simulink model "Multi_FW_formation_control_wind"  (R2023b)
settings: Solver=FixedStepAuto  StartTime=0.0  StopTime=70  FixedStep=0.001  RelTol=1e-3
undefined symbols (not defined in the file or in its folder): fc, hc, lc
libraries: Fixed_Wing x4, simulink x1
settings Model: Creator=TigerWuu  LastModifiedBy=NCS
settings SolverCC: MaxConsecutiveMinStep=10  ZeroCrossAlgorithm=Adaptive  EnableFixedStepZeroCrossing=on
settings OptimizationCC: EnhancedBackFolding=on  PassReuseOutputArgsAs=Individual arguments  ZeroExternalMemoryAtStartup=off  ZeroInternalMemoryAtStartup=off  MaxStackSize=64  OptimizeBlockOrder=speed  DifferentSizesBufferReuse=on  OptimizationCustomize=off  EfficientTunableParamExpr=on
settings DebuggingCC: IgnoredZcDiagnostic=none  ParameterTunabilityLossMsg=error  UnconnectedInputMsg=warning  UnconnectedOutputMsg=warning  UnconnectedLineMsg=warning  UnderSpecifiedDimensionMsg=warning
settings HardwareCC: UseEmbeddedCoderFeatures=off
settings ModelReferenceCC: EnableRefExpFcnMdlSchedulingChecks=on
settings SFSimCC: MATLABDynamicMemAlloc=off
settings RTWCC: Description=Embedded Coder  SystemTargetFile=ert.tlc  HardwareBoard=Robot Operating System 2 (ROS 2)  TLCOptions="-aInlineSetEventsForThisBaseRateFcn=TLC_FALSE -aSuppressMultiTaskScheduler=TLC_FALSE  -aRateBasedStepFcn=0"  TemplateMakefile=ert_default_tmf  Toolchain=Colcon Tools  TargetLang=C++  DLArmComputeVersion=19.05
settings CodeAppCC: ForceParamTrailComments=on  IgnoreCustomStorageClasses=off  OperatorAnnotations=on  SimulinkDataObjDesc=on  SFDataObjDesc=on  InsertBlockDesc=on
settings ERTTargetCC: CodeInterfacePackaging=C++ class  SupportNonInlinedSFcns=on  RootIOFormat=Structure reference

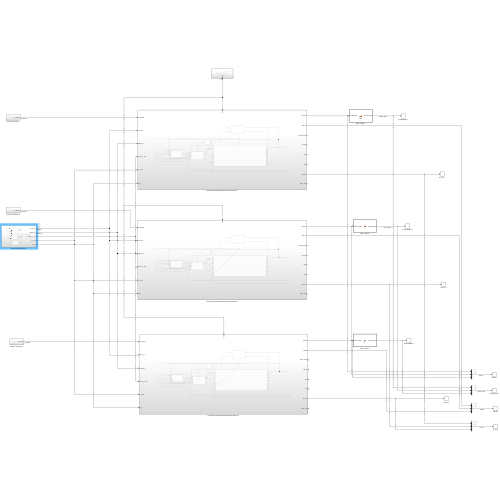
[thumbnail: Simulink's stored preview of the top-level diagram]
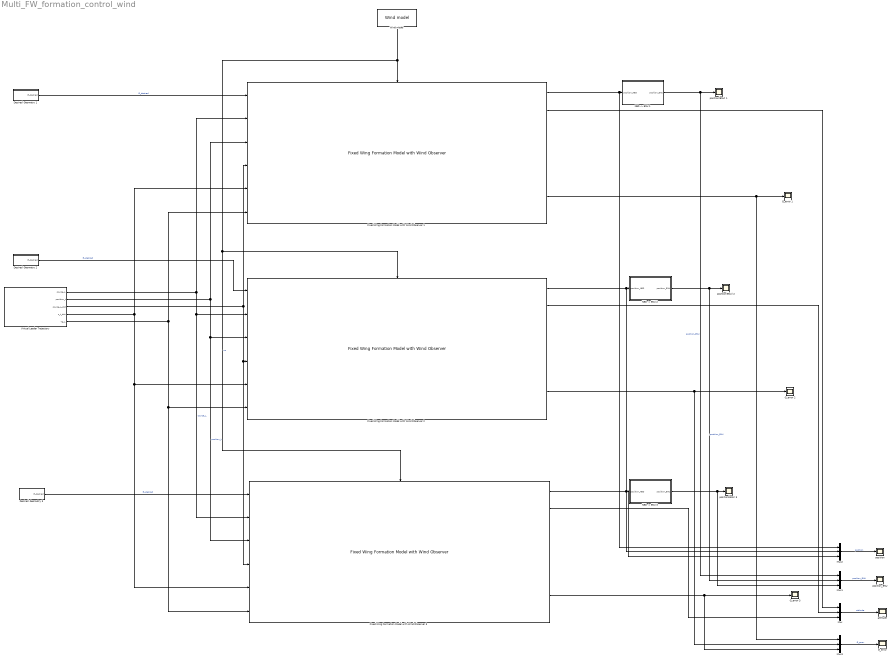
== system Multi_FW_formation_control_wind ==
  Desired  Geometry 1 : Subsystem
  Desired  Geometry 2 : Subsystem
  Desired  Geometry 3 : Subsystem
  Fixed Wing Formation Model with Wind Observer 1 : Fixed_Wing/Fixed Wing Formation Model with Wind Observer  SystemSampleTime=-1  VariantActivationTime=update diagram  AllowFlexibleInterface=on  Latency=0  AutoFrameSizeCalculation=off
      settings: SourceProductName=Fixed-Wing Model  PortSchema="{\"entries\":[{\"content\":{\"sides\":[{\"content\":{\"connectorIds\":[\"In1\",\"In2\",\"In3\",\"In4\",\"In5\",\"In6\"]},\"type\":\"ConnectorPlacement.EquallySpacedRectSide\",\"uuid\":\"527b8280-b7bb-4bbf-b75e-797629a1d02f\"},{\"content\":{\"connectorIds\":[\"Out1\",\"Out2\",\"Out3\",\"Out4\",\"Out5\",\"Out6\",\"Out7\",\"Out8\"],\"side\":\"RIGHT\"},\"type\":\"ConnectorPlacement.EquallySpacedRectSide\",\"uuid\":\"83651618-4cce-4797-8c5d-5752aadadd0e\"},{\"content\":{\"connectorIds\":[\"In7\"],\"side\":\"TOP\"},\"type\":\"ConnectorPlacement.EquallySpacedRectSide\",\"uuid\":\"91f129b3-c1c6-46ff-9e73-d368da7d167a\"}]},\"type\":\"ConnectorPlacement.EquallySpacedConnector\",\"uuid\":\"d5eae0c8-1f9e-4313-b74c-0f7e22e43491\"}],\"packageUris\":[\"http://schema.mathworks.com/mf0/Connector/R2020b\"],\"version\":\"1.0\"}"
  Fixed Wing Formation Model with Wind Observer 2 : Fixed_Wing/Fixed Wing Formation Model with Wind Observer  SystemSampleTime=-1  VariantActivationTime=update diagram  AllowFlexibleInterface=on  Latency=0  AutoFrameSizeCalculation=off
      settings: SourceProductName=Fixed-Wing Model  PortSchema="{\"entries\":[{\"content\":{\"sides\":[{\"content\":{\"connectorIds\":[\"In1\",\"In2\",\"In3\",\"In4\",\"In5\",\"In6\"]},\"type\":\"ConnectorPlacement.EquallySpacedRectSide\",\"uuid\":\"527b8280-b7bb-4bbf-b75e-797629a1d02f\"},{\"content\":{\"connectorIds\":[\"Out1\",\"Out2\",\"Out3\",\"Out4\",\"Out5\",\"Out6\",\"Out7\",\"Out8\"],\"side\":\"RIGHT\"},\"type\":\"ConnectorPlacement.EquallySpacedRectSide\",\"uuid\":\"83651618-4cce-4797-8c5d-5752aadadd0e\"},{\"content\":{\"connectorIds\":[\"In7\"],\"side\":\"TOP\"},\"type\":\"ConnectorPlacement.EquallySpacedRectSide\",\"uuid\":\"91f129b3-c1c6-46ff-9e73-d368da7d167a\"}]},\"type\":\"ConnectorPlacement.EquallySpacedConnector\",\"uuid\":\"d5eae0c8-1f9e-4313-b74c-0f7e22e43491\"}],\"packageUris\":[\"http://schema.mathworks.com/mf0/Connector/R2020b\"],\"version\":\"1.0\"}"
  Fixed Wing Formation Model with Wind Observer 3 : Fixed_Wing/Fixed Wing Formation Model with Wind Observer  SystemSampleTime=-1  VariantActivationTime=update diagram  AllowFlexibleInterface=on  Latency=0  AutoFrameSizeCalculation=off
      settings: SourceProductName=Fixed-Wing Model  PortSchema="{\"entries\":[{\"content\":{\"sides\":[{\"content\":{\"connectorIds\":[\"In1\",\"In2\",\"In3\",\"In4\",\"In5\",\"In6\"]},\"type\":\"ConnectorPlacement.EquallySpacedRectSide\",\"uuid\":\"527b8280-b7bb-4bbf-b75e-797629a1d02f\"},{\"content\":{\"connectorIds\":[\"Out1\",\"Out2\",\"Out3\",\"Out4\",\"Out5\",\"Out6\",\"Out7\",\"Out8\"],\"side\":\"RIGHT\"},\"type\":\"ConnectorPlacement.EquallySpacedRectSide\",\"uuid\":\"83651618-4cce-4797-8c5d-5752aadadd0e\"},{\"content\":{\"connectorIds\":[\"In7\"],\"side\":\"TOP\"},\"type\":\"ConnectorPlacement.EquallySpacedRectSide\",\"uuid\":\"91f129b3-c1c6-46ff-9e73-d368da7d167a\"}]},\"type\":\"ConnectorPlacement.EquallySpacedConnector\",\"uuid\":\"d5eae0c8-1f9e-4313-b74c-0f7e22e43491\"}],\"packageUris\":[\"http://schema.mathworks.com/mf0/Connector/R2020b\"],\"version\":\"1.0\"}"
  G_error : Scope
  G_error 1 : Scope
  G_error 2 : Scope
  G_error 3 : Scope
  Mux{,1..3} (4 alike) : Mux  Inputs=3
  "NED -> ENU 1" : MATLAB Function  TreatAsAtomicUnit=on
  "NED -> ENU 2" : MATLAB Function  TreatAsAtomicUnit=on
  "NED -> ENU 3" : MATLAB Function  TreatAsAtomicUnit=on
  Virtual Leader Trajectory : Subsystem
  Wind model : Fixed_Wing/Wind model  SystemSampleTime=-1  VariantActivationTime=update diagram  AllowFlexibleInterface=on  Latency=0  AutoFrameSizeCalculation=off
      settings: SourceProductName=Fixed-Wing Model  PortSchema="{\"entries\":[{\"content\":{\"sides\":[{\"content\":{},\"type\":\"ConnectorPlacement.EquallySpacedRectSide\",\"uuid\":\"19ef0eb7-c626-45ec-b76b-8668fc024824\"},{\"content\":{\"side\":\"RIGHT\"},\"type\":\"ConnectorPlacement.EquallySpacedRectSide\",\"uuid\":\"89e72569-ab94-4162-a6e2-b425ef08f724\"},{\"content\":{\"side\":\"TOP\"},\"type\":\"ConnectorPlacement.EquallySpacedRectSide\",\"uuid\":\"6d9409e9-6822-4cd9-902f-e5665cb68433\"},{\"content\":{\"connectorIds\":[\"Out1\"],\"side\":\"BOTTOM\"},\"type\":\"ConnectorPlacement.EquallySpacedRectSide\",\"uuid\":\"39a83352-0924-44fa-be5d-94a7c28bbbf3\"}]},\"type\":\"ConnectorPlacement.EquallySpacedConnector\",\"uuid\":\"6cf6ae00-ef23-42a2-99b2-ca60e191fb03\"}],\"packageUris\":[\"http://schema.mathworks.com/mf0/Connector/R2020b\"],\"version\":\"1.0\"}"
  attitude : Scope
  position : Scope
  position(ENU) 1 : Scope
  position(ENU) 2 : Scope
  position(ENU) 3 : Scope
  position_ENU : Scope
  wires:
  "NED -> ENU 1"/1(position_ENU) -> Mux1/1, position(ENU) 1/1  "position_ENU"
  Desired  Geometry 1/1(G_desired) -> Fixed Wing Formation Model with Wind Observer 1/1  "G_desired"
  Virtual Leader Trajectory/1(course_L) -> Fixed Wing Formation Model with Wind Observer 2/2, Fixed Wing Formation Model with Wind Observer 3/2, Fixed Wing Formation Model with Wind Observer 1/2  "course_L"
  Virtual Leader Trajectory/2(position_L) -> Fixed Wing Formation Model with Wind Observer 2/3, Fixed Wing Formation Model with Wind Observer 3/3, Fixed Wing Formation Model with Wind Observer 1/3  "position_L"
  Virtual Leader Trajectory/3(course_L_dot) -> Fixed Wing Formation Model with Wind Observer 2/4, Fixed Wing Formation Model with Wind Observer 3/4, Fixed Wing Formation Model with Wind Observer 1/4
  Virtual Leader Trajectory/4(z_L_dot) -> Fixed Wing Formation Model with Wind Observer 2/5, Fixed Wing Formation Model with Wind Observer 3/5, Fixed Wing Formation Model with Wind Observer 1/5
  Virtual Leader Trajectory/5(Vg_L) -> Fixed Wing Formation Model with Wind Observer 2/6, Fixed Wing Formation Model with Wind Observer 3/6, Fixed Wing Formation Model with Wind Observer 1/6
  Wind model/1 -> Fixed Wing Formation Model with Wind Observer 1/7, Fixed Wing Formation Model with Wind Observer 2/7, Fixed Wing Formation Model with Wind Observer 3/7  "ws"
  Fixed Wing Formation Model with Wind Observer 1/1 -> Mux2/1, "NED -> ENU 1"/1(position_NED)
  Desired  Geometry 2/1(G_desired) -> Fixed Wing Formation Model with Wind Observer 2/1  "G_desired"
  "NED -> ENU 2"/1(position_ENU) -> Mux1/2, position(ENU) 2/1  "position_ENU"
  Fixed Wing Formation Model with Wind Observer 2/1 -> Mux2/2, "NED -> ENU 2"/1(position_NED)
  Fixed Wing Formation Model with Wind Observer 2/7 -> Mux3/2, G_error 2/1
  Desired  Geometry 3/1(G_desired) -> Fixed Wing Formation Model with Wind Observer 3/1  "G_desired"
  "NED -> ENU 3"/1(position_ENU) -> Mux1/3, position(ENU) 3/1
  Fixed Wing Formation Model with Wind Observer 3/1 -> Mux2/3, "NED -> ENU 3"/1(position_NED)
  Fixed Wing Formation Model with Wind Observer 3/7 -> Mux3/3, G_error 3/1
  Fixed Wing Formation Model with Wind Observer 1/2 -> Mux/1
  Fixed Wing Formation Model with Wind Observer 2/2 -> Mux/2
  Fixed Wing Formation Model with Wind Observer 3/2 -> Mux/3
  Fixed Wing Formation Model with Wind Observer 1/7 -> Mux3/1, G_error 1/1
  Mux2/1 -> position/1  "position"
  Mux1/1 -> position_ENU/1  "position_ENU"
  Mux/1 -> attitude/1  "attitude"
  Mux3/1 -> G_error/1  "G_error"

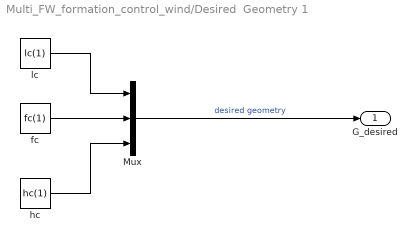
== system Multi_FW_formation_control_wind/Desired  Geometry 1 ==
  Mux : Mux  Inputs=3
  fc : Constant  Value=fc(1)
  hc : Constant  Value=hc(1)
  lc : Constant  Value=lc(1)
  G_desired : Outport
  wires:
  Mux/1 -> G_desired/1  "desired geometry"
  lc/1 -> Mux/1
  fc/1 -> Mux/2
  hc/1 -> Mux/3

== system Multi_FW_formation_control_wind/Desired  Geometry 2 ==
  Mux : Mux  Inputs=3
  fc : Constant  Value=fc(2)
  hc : Constant  Value=hc(2)
  lc : Constant  Value=lc(2)
  G_desired : Outport
  wires:
  Mux/1 -> G_desired/1  "desired geometry"
  lc/1 -> Mux/1
  fc/1 -> Mux/2
  hc/1 -> Mux/3

== system Multi_FW_formation_control_wind/Desired  Geometry 3 ==
  Mux : Mux  Inputs=3
  fc : Constant  Value=fc(3)
  hc : Constant  Value=hc(3)
  lc : Constant  Value=lc(3)
  G_desired : Outport
  wires:
  Mux/1 -> G_desired/1  "desired geometry"
  lc/1 -> Mux/1
  fc/1 -> Mux/2
  hc/1 -> Mux/3

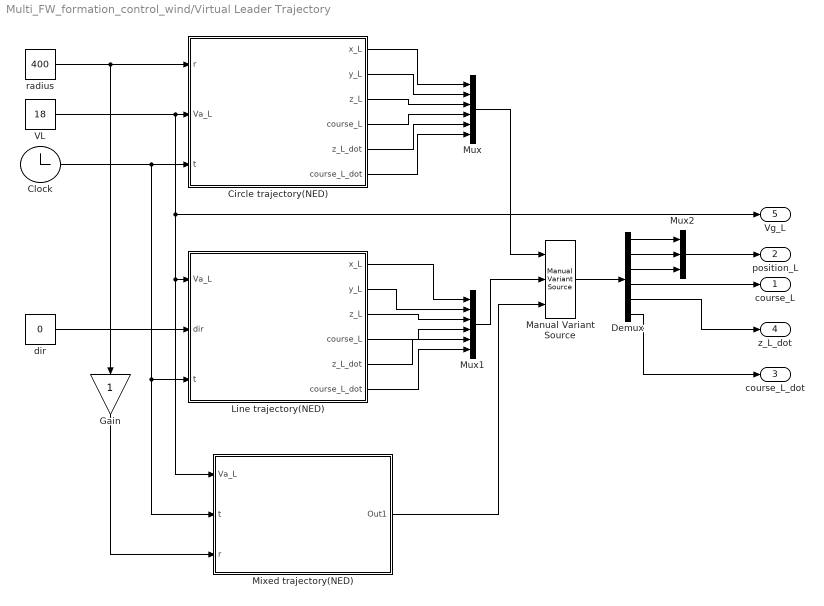
== system Multi_FW_formation_control_wind/Virtual Leader Trajectory ==
  Circle trajectory(NED) : MATLAB Function  TreatAsAtomicUnit=on
  Clock : Clock
  Demux : Demux  Outputs=6
  Gain : Gain
  Line trajectory(NED) : MATLAB Function  TreatAsAtomicUnit=on
  Manual Variant Source : simulink/Signal Routing/Manual Variant Source  NumChoices=3  LabelModeActiveChoice=V_2
  Mixed trajectory(NED) : Subsystem
  Mux : Mux  Inputs=6
  Mux1 : Mux  Inputs=6
  Mux2 : Mux  Inputs=3
  VL : Constant  Value=18
  dir : Constant  Value=0
  radius : Constant  Value=400
  course_L : Outport
  position_L : Outport  Port=2
  course_L_dot : Outport  Port=3
  z_L_dot : Outport  Port=4
  Vg_L : Outport  Port=5
  wires:
  radius/1 -> Circle trajectory(NED)/1(r), Gain/1
  VL/1 -> Vg_L/1, Mixed trajectory(NED)/1(Va_L), Line trajectory(NED)/1(Va_L), Circle trajectory(NED)/2(Va_L)
  Clock/1 -> Mixed trajectory(NED)/2(t), Line trajectory(NED)/3(t), Circle trajectory(NED)/3(t)
  Mux/1 -> Manual Variant Source/1
  Circle trajectory(NED)/1(x_L) -> Mux/1
  Circle trajectory(NED)/2(y_L) -> Mux/2
  Circle trajectory(NED)/3(z_L) -> Mux/3
  Line trajectory(NED)/1(x_L) -> Mux1/1
  Line trajectory(NED)/2(y_L) -> Mux1/2
  Line trajectory(NED)/3(z_L) -> Mux1/3
  Line trajectory(NED)/4(course_L) -> Mux1/4
  Mux1/1 -> Manual Variant Source/2
  Manual Variant Source/1 -> Demux/1
  Demux/1 -> Mux2/1
  Demux/2 -> Mux2/2
  Demux/3 -> Mux2/3
  Mux2/1 -> position_L/1
  Circle trajectory(NED)/6(course_L_dot) -> Mux/6
  Line trajectory(NED)/6(course_L_dot) -> Mux1/6
  Line trajectory(NED)/5(z_L_dot) -> Mux1/5
  Demux/4 -> course_L/1
  Demux/5 -> z_L_dot/1
  Demux/6 -> course_L_dot/1
  Circle trajectory(NED)/4(course_L) -> Mux/4
  Circle trajectory(NED)/5(z_L_dot) -> Mux/5
  Gain/1 -> Mixed trajectory(NED)/3(r)
  Mixed trajectory(NED)/1(Out1) -> Manual Variant Source/3
  dir/1 -> Line trajectory(NED)/2(dir)

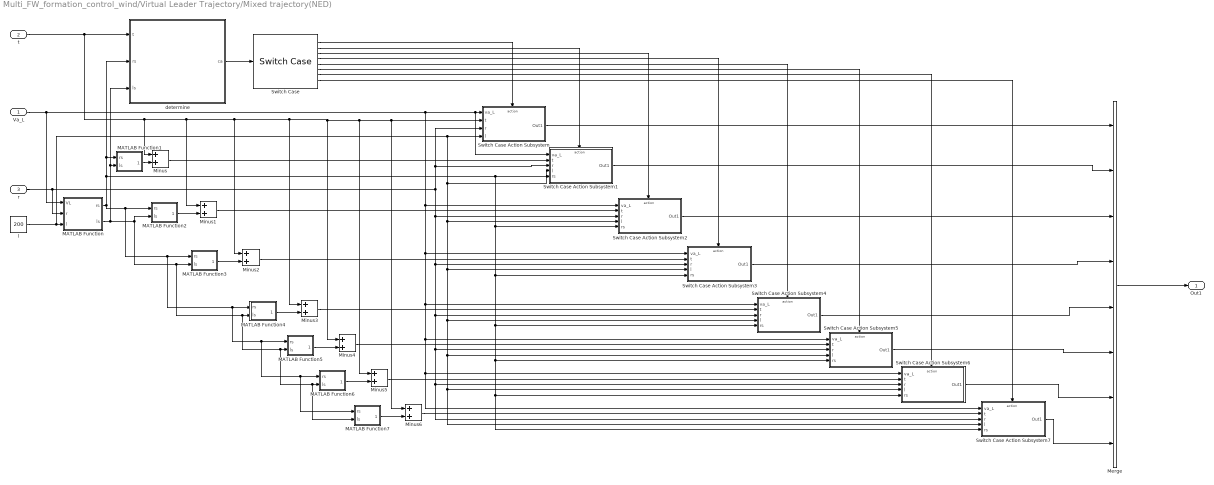
== system Multi_FW_formation_control_wind/Virtual Leader Trajectory/Mixed trajectory(NED) ==
  Va_L : Inport
  t : Inport  Port=2
  r : Inport  Port=3
  MATLAB Function : MATLAB Function  TreatAsAtomicUnit=on
  MATLAB Function1 : MATLAB Function  TreatAsAtomicUnit=on
  MATLAB Function2 : MATLAB Function  TreatAsAtomicUnit=on
  MATLAB Function3 : MATLAB Function  TreatAsAtomicUnit=on
  MATLAB Function4 : MATLAB Function  TreatAsAtomicUnit=on
  MATLAB Function5 : MATLAB Function  TreatAsAtomicUnit=on
  MATLAB Function6 : MATLAB Function  TreatAsAtomicUnit=on
  MATLAB Function7 : MATLAB Function  TreatAsAtomicUnit=on
  Merge : Merge  Inputs=8
  Minus{,1..6} (7 alike) : Sum
  Switch Case : SwitchCase  CaseConditions={1,2,3,4,5,6,7,8}  ShowDefaultCase=off
  Switch Case Action Subsystem : Subsystem  TreatAsAtomicUnit=on
  Switch Case Action Subsystem1 : Subsystem  TreatAsAtomicUnit=on
  Switch Case Action Subsystem2 : Subsystem  TreatAsAtomicUnit=on
  Switch Case Action Subsystem3 : Subsystem  TreatAsAtomicUnit=on
  Switch Case Action Subsystem4 : Subsystem  TreatAsAtomicUnit=on
  Switch Case Action Subsystem5 : Subsystem  TreatAsAtomicUnit=on
  Switch Case Action Subsystem6 : Subsystem  TreatAsAtomicUnit=on
  Switch Case Action Subsystem7 : Subsystem  TreatAsAtomicUnit=on
  determine : MATLAB Function  TreatAsAtomicUnit=on
  l : Constant  Value=200
  Out1 : Outport
  wires:
  determine/1(ca) -> Switch Case/1
  Switch Case/1 -> Switch Case Action Subsystem/Action
  MATLAB Function1/1(offset) -> Minus/2
  Switch Case/2 -> Switch Case Action Subsystem1/Action
  r/1 -> Switch Case Action Subsystem6/3(r), Switch Case Action Subsystem7/3(r), Switch Case Action Subsystem5/3(r), Switch Case Action Subsystem4/3(r), Switch Case Action Subsystem3/3(r), Switch Case Action Subsystem2/3(r), Switch Case Action Subsystem/3(r), Switch Case Action Subsystem1/3(r), MATLAB Function/2(r)
  MATLAB Function2/1(offset) -> Minus1/2
  Minus1/1 -> Switch Case Action Subsystem2/2(t)
  Switch Case/3 -> Switch Case Action Subsystem2/Action
  Switch Case/4 -> Switch Case Action Subsystem3/Action
  Minus/1 -> Switch Case Action Subsystem1/2(t)
  MATLAB Function3/1(offset) -> Minus2/2
  Minus2/1 -> Switch Case Action Subsystem3/2(t)
  Va_L/1 -> Switch Case Action Subsystem1/1(va_L), Switch Case Action Subsystem/1(va_L), Switch Case Action Subsystem4/1(va_L), Switch Case Action Subsystem5/1(va_L), Switch Case Action Subsystem6/1(va_L), Switch Case Action Subsystem7/1(va_L), Switch Case Action Subsystem3/1(va_L), Switch Case Action Subsystem2/1(va_L), MATLAB Function/1(VL)
  Minus3/1 -> Switch Case Action Subsystem4/2(t)
  Switch Case/5 -> Switch Case Action Subsystem4/Action
  MATLAB Function4/1(offset) -> Minus3/2
  Switch Case/6 -> Switch Case Action Subsystem5/Action
  MATLAB Function5/1(offset) -> Minus4/2
  Minus4/1 -> Switch Case Action Subsystem5/2(t)
  Switch Case/7 -> Switch Case Action Subsystem6/Action
  MATLAB Function6/1(offset) -> Minus5/2
  Minus5/1 -> Switch Case Action Subsystem6/2(t)
  Switch Case/8 -> Switch Case Action Subsystem7/Action
  t/1 -> Minus/1, Minus1/1, Minus2/1, Minus3/1, Minus4/1, Minus5/1, Minus6/1, Switch Case Action Subsystem/2(t), determine/1(t)
  Minus6/1 -> Switch Case Action Subsystem7/2(t)
  MATLAB Function7/1(offset) -> Minus6/2
  Switch Case Action Subsystem/1(Out1) -> Merge/1
  Switch Case Action Subsystem1/1(Out1) -> Merge/2
  Switch Case Action Subsystem2/1(Out1) -> Merge/3
  Switch Case Action Subsystem3/1(Out1) -> Merge/4
  Switch Case Action Subsystem4/1(Out1) -> Merge/5
  Switch Case Action Subsystem5/1(Out1) -> Merge/6
  Switch Case Action Subsystem6/1(Out1) -> Merge/7
  Switch Case Action Subsystem7/1(Out1) -> Merge/8
  Merge/1 -> Out1/1
  l/1 -> Switch Case Action Subsystem/4(l), Switch Case Action Subsystem5/4(l), Switch Case Action Subsystem6/4(l), Switch Case Action Subsystem7/4(l), Switch Case Action Subsystem4/4(l), Switch Case Action Subsystem3/4(l), Switch Case Action Subsystem2/4(l), Switch Case Action Subsystem1/4(l), MATLAB Function/3(l)
  MATLAB Function/1(rs) -> MATLAB Function7/1(rs), MATLAB Function6/1(rs), MATLAB Function5/1(rs), MATLAB Function4/1(rs), MATLAB Function3/1(rs), MATLAB Function2/1(rs), MATLAB Function1/1(rs), determine/2(rs), Switch Case Action Subsystem4/5(rs), Switch Case Action Subsystem5/5(rs), Switch Case Action Subsystem6/5(rs), Switch Case Action Subsystem7/5(rs), Switch Case Action Subsystem3/5(rs), Switch Case Action Subsystem2/5(rs), Switch Case Action Subsystem1/5(rs)
  MATLAB Function/2(ls) -> MATLAB Function7/2(ls), MATLAB Function6/2(ls), MATLAB Function5/2(ls), MATLAB Function4/2(ls), MATLAB Function3/2(ls), MATLAB Function2/2(ls), MATLAB Function1/2(ls), determine/3(ls)

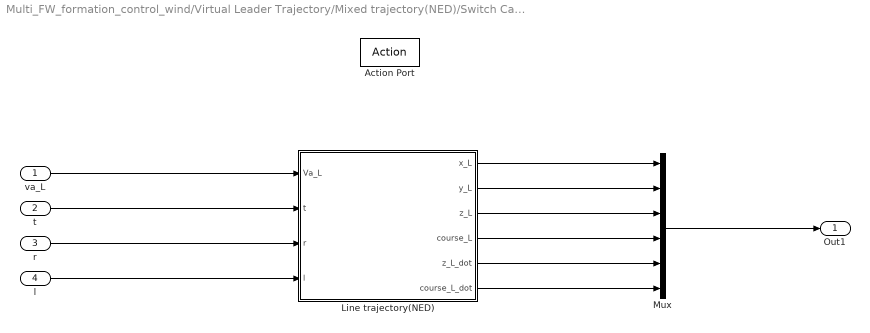
== system Multi_FW_formation_control_wind/Virtual Leader Trajectory/Mixed trajectory(NED)/Switch Case Action Subsystem ==
  va_L : Inport
  t : Inport  Port=2
  r : Inport  Port=3
  l : Inport  Port=4
  Action Port : ActionPort
  Line trajectory(NED) : MATLAB Function  TreatAsAtomicUnit=on
  Mux : Mux  Inputs=6
  Out1 : Outport
  wires:
  t/1 -> Line trajectory(NED)/2(t)
  va_L/1 -> Line trajectory(NED)/1(Va_L)
  Line trajectory(NED)/6(course_L_dot) -> Mux/6
  Line trajectory(NED)/5(z_L_dot) -> Mux/5
  Line trajectory(NED)/4(course_L) -> Mux/4
  Line trajectory(NED)/3(z_L) -> Mux/3
  Line trajectory(NED)/2(y_L) -> Mux/2
  Line trajectory(NED)/1(x_L) -> Mux/1
  Mux/1 -> Out1/1
  r/1 -> Line trajectory(NED)/3(r)
  l/1 -> Line trajectory(NED)/4(l)

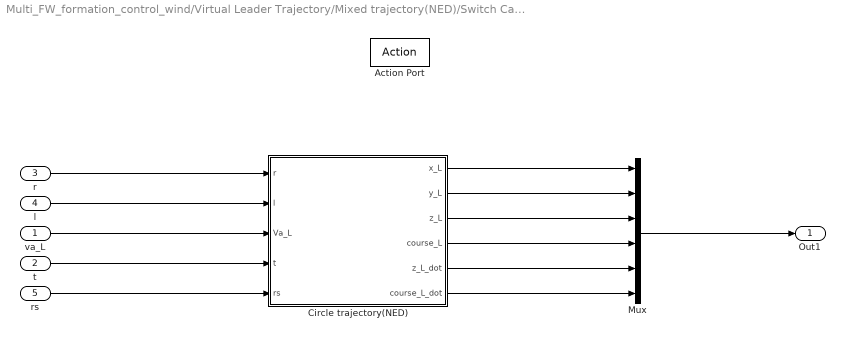
== system Multi_FW_formation_control_wind/Virtual Leader Trajectory/Mixed trajectory(NED)/Switch Case Action Subsystem1 ==
  va_L : Inport
  t : Inport  Port=2
  r : Inport  Port=3
  l : Inport  Port=4
  rs : Inport  Port=5
  Action Port : ActionPort
  Circle trajectory(NED) : MATLAB Function  TreatAsAtomicUnit=on
  Mux : Mux  Inputs=6
  Out1 : Outport
  wires:
  t/1 -> Circle trajectory(NED)/4(t)
  va_L/1 -> Circle trajectory(NED)/3(Va_L)
  Circle trajectory(NED)/6(course_L_dot) -> Mux/6
  Circle trajectory(NED)/5(z_L_dot) -> Mux/5
  Circle trajectory(NED)/4(course_L) -> Mux/4
  Circle trajectory(NED)/3(z_L) -> Mux/3
  Circle trajectory(NED)/2(y_L) -> Mux/2
  Circle trajectory(NED)/1(x_L) -> Mux/1
  Mux/1 -> Out1/1
  r/1 -> Circle trajectory(NED)/1(r)
  l/1 -> Circle trajectory(NED)/2(l)
  rs/1 -> Circle trajectory(NED)/5(rs)

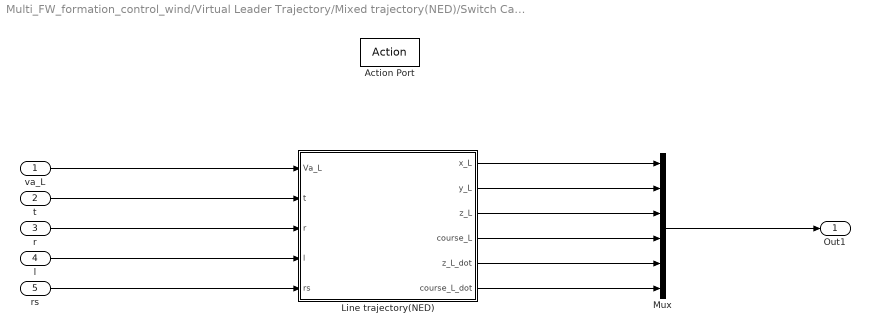
== system Multi_FW_formation_control_wind/Virtual Leader Trajectory/Mixed trajectory(NED)/Switch Case Action Subsystem2 ==
  va_L : Inport
  t : Inport  Port=2
  r : Inport  Port=3
  l : Inport  Port=4
  rs : Inport  Port=5
  Action Port : ActionPort
  Line trajectory(NED) : MATLAB Function  TreatAsAtomicUnit=on
  Mux : Mux  Inputs=6
  Out1 : Outport
  wires:
  t/1 -> Line trajectory(NED)/2(t)
  va_L/1 -> Line trajectory(NED)/1(Va_L)
  Line trajectory(NED)/6(course_L_dot) -> Mux/6
  Line trajectory(NED)/5(z_L_dot) -> Mux/5
  Line trajectory(NED)/4(course_L) -> Mux/4
  Line trajectory(NED)/3(z_L) -> Mux/3
  Line trajectory(NED)/2(y_L) -> Mux/2
  Line trajectory(NED)/1(x_L) -> Mux/1
  Mux/1 -> Out1/1
  rs/1 -> Line trajectory(NED)/5(rs)
  l/1 -> Line trajectory(NED)/4(l)
  r/1 -> Line trajectory(NED)/3(r)

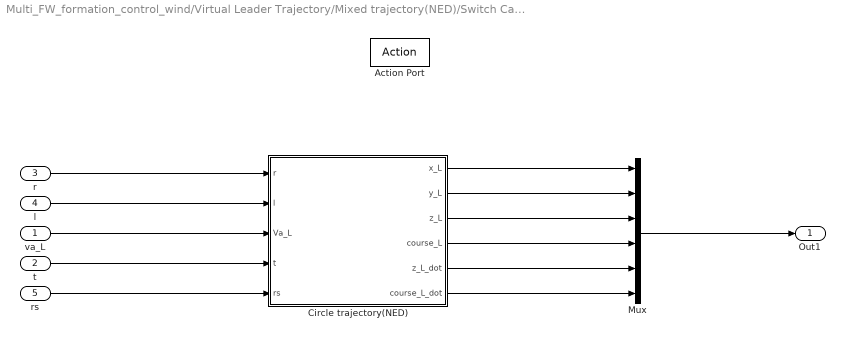
== system Multi_FW_formation_control_wind/Virtual Leader Trajectory/Mixed trajectory(NED)/Switch Case Action Subsystem3 ==
  va_L : Inport
  t : Inport  Port=2
  r : Inport  Port=3
  l : Inport  Port=4
  rs : Inport  Port=5
  Action Port : ActionPort
  Circle trajectory(NED) : MATLAB Function  TreatAsAtomicUnit=on
  Mux : Mux  Inputs=6
  Out1 : Outport
  wires:
  t/1 -> Circle trajectory(NED)/4(t)
  va_L/1 -> Circle trajectory(NED)/3(Va_L)
  Circle trajectory(NED)/6(course_L_dot) -> Mux/6
  Circle trajectory(NED)/5(z_L_dot) -> Mux/5
  Circle trajectory(NED)/4(course_L) -> Mux/4
  Circle trajectory(NED)/3(z_L) -> Mux/3
  Circle trajectory(NED)/2(y_L) -> Mux/2
  Circle trajectory(NED)/1(x_L) -> Mux/1
  Mux/1 -> Out1/1
  r/1 -> Circle trajectory(NED)/1(r)
  rs/1 -> Circle trajectory(NED)/5(rs)
  l/1 -> Circle trajectory(NED)/2(l)

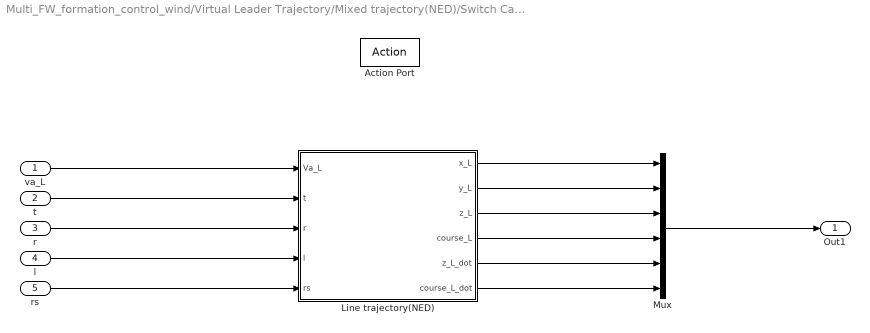
== system Multi_FW_formation_control_wind/Virtual Leader Trajectory/Mixed trajectory(NED)/Switch Case Action Subsystem4 ==
  va_L : Inport
  t : Inport  Port=2
  r : Inport  Port=3
  l : Inport  Port=4
  rs : Inport  Port=5
  Action Port : ActionPort
  Line trajectory(NED) : MATLAB Function  TreatAsAtomicUnit=on
  Mux : Mux  Inputs=6
  Out1 : Outport
  wires:
  t/1 -> Line trajectory(NED)/2(t)
  va_L/1 -> Line trajectory(NED)/1(Va_L)
  Line trajectory(NED)/6(course_L_dot) -> Mux/6
  Line trajectory(NED)/5(z_L_dot) -> Mux/5
  Line trajectory(NED)/4(course_L) -> Mux/4
  Line trajectory(NED)/3(z_L) -> Mux/3
  Line trajectory(NED)/2(y_L) -> Mux/2
  Line trajectory(NED)/1(x_L) -> Mux/1
  Mux/1 -> Out1/1
  r/1 -> Line trajectory(NED)/3(r)
  l/1 -> Line trajectory(NED)/4(l)
  rs/1 -> Line trajectory(NED)/5(rs)

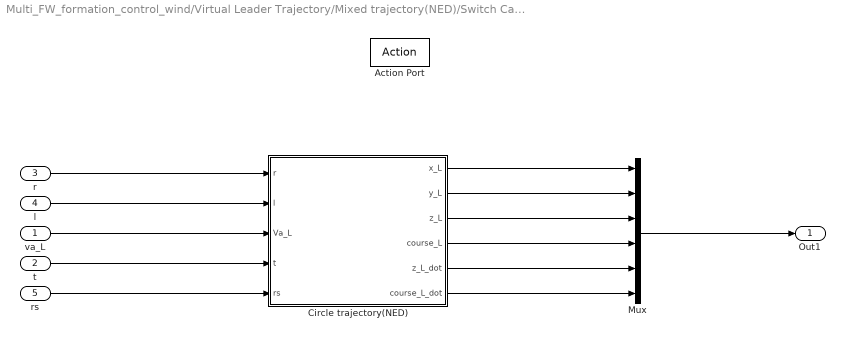
== system Multi_FW_formation_control_wind/Virtual Leader Trajectory/Mixed trajectory(NED)/Switch Case Action Subsystem5 ==
  va_L : Inport
  t : Inport  Port=2
  r : Inport  Port=3
  l : Inport  Port=4
  rs : Inport  Port=5
  Action Port : ActionPort
  Circle trajectory(NED) : MATLAB Function  TreatAsAtomicUnit=on
  Mux : Mux  Inputs=6
  Out1 : Outport
  wires:
  t/1 -> Circle trajectory(NED)/4(t)
  va_L/1 -> Circle trajectory(NED)/3(Va_L)
  Circle trajectory(NED)/6(course_L_dot) -> Mux/6
  Circle trajectory(NED)/5(z_L_dot) -> Mux/5
  Circle trajectory(NED)/4(course_L) -> Mux/4
  Circle trajectory(NED)/3(z_L) -> Mux/3
  Circle trajectory(NED)/2(y_L) -> Mux/2
  Circle trajectory(NED)/1(x_L) -> Mux/1
  Mux/1 -> Out1/1
  r/1 -> Circle trajectory(NED)/1(r)
  rs/1 -> Circle trajectory(NED)/5(rs)
  l/1 -> Circle trajectory(NED)/2(l)

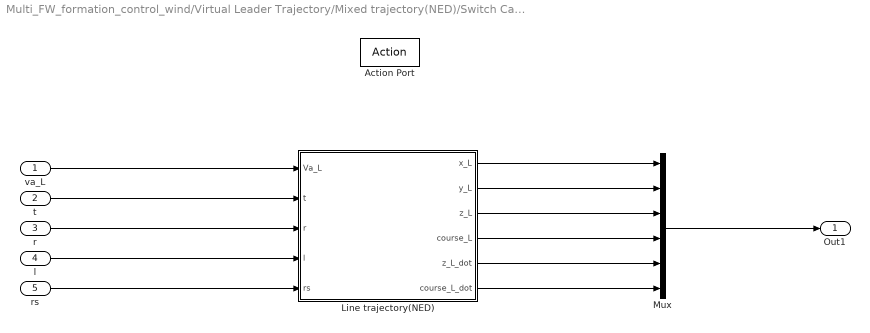
== system Multi_FW_formation_control_wind/Virtual Leader Trajectory/Mixed trajectory(NED)/Switch Case Action Subsystem6 ==
  va_L : Inport
  t : Inport  Port=2
  r : Inport  Port=3
  l : Inport  Port=4
  rs : Inport  Port=5
  Action Port : ActionPort
  Line trajectory(NED) : MATLAB Function  TreatAsAtomicUnit=on
  Mux : Mux  Inputs=6
  Out1 : Outport
  wires:
  t/1 -> Line trajectory(NED)/2(t)
  va_L/1 -> Line trajectory(NED)/1(Va_L)
  Line trajectory(NED)/6(course_L_dot) -> Mux/6
  Line trajectory(NED)/5(z_L_dot) -> Mux/5
  Line trajectory(NED)/4(course_L) -> Mux/4
  Line trajectory(NED)/3(z_L) -> Mux/3
  Line trajectory(NED)/2(y_L) -> Mux/2
  Line trajectory(NED)/1(x_L) -> Mux/1
  Mux/1 -> Out1/1
  r/1 -> Line trajectory(NED)/3(r)
  l/1 -> Line trajectory(NED)/4(l)
  rs/1 -> Line trajectory(NED)/5(rs)

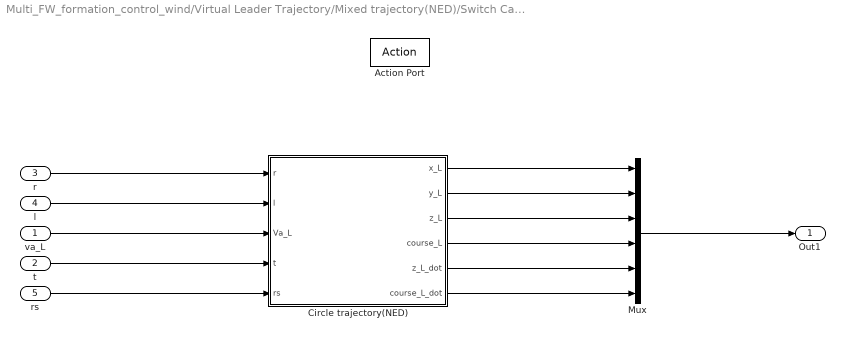
== system Multi_FW_formation_control_wind/Virtual Leader Trajectory/Mixed trajectory(NED)/Switch Case Action Subsystem7 ==
  va_L : Inport
  t : Inport  Port=2
  r : Inport  Port=3
  l : Inport  Port=4
  rs : Inport  Port=5
  Action Port : ActionPort
  Circle trajectory(NED) : MATLAB Function  TreatAsAtomicUnit=on
  Mux : Mux  Inputs=6
  Out1 : Outport
  wires:
  t/1 -> Circle trajectory(NED)/4(t)
  va_L/1 -> Circle trajectory(NED)/3(Va_L)
  Circle trajectory(NED)/6(course_L_dot) -> Mux/6
  Circle trajectory(NED)/5(z_L_dot) -> Mux/5
  Circle trajectory(NED)/4(course_L) -> Mux/4
  Circle trajectory(NED)/3(z_L) -> Mux/3
  Circle trajectory(NED)/2(y_L) -> Mux/2
  Circle trajectory(NED)/1(x_L) -> Mux/1
  Mux/1 -> Out1/1
  r/1 -> Circle trajectory(NED)/1(r)
  l/1 -> Circle trajectory(NED)/2(l)
  rs/1 -> Circle trajectory(NED)/5(rs)

== matlab function Multi_FW_formation_control_wind/Virtual Leader Trajectory/Mixed trajectory(NED)/Switch Case Action Subsystem1/Circle trajectory(NED) ==
  data: x_L output; y_L output; z_L output; course_L output; z_L_dot output; course_L_dot output; r input; l input; Va_L input; t input; rs input
  function [x_L, y_L, z_L, course_L, z_L_dot, course_L_dot] = trajectory_generation(r,l,Va_L, t, rs)
    t1 = t - rs;
    climbing_rate = -2; % 3D
    Va_Lp = sqrt(Va_L^2-climbing_rate^2);
    omega = Va_Lp/r; % rad/s
    x_L = l/2+r*sin(omega*t);
    y_L = -l/2+r*cos(omega*t);
    z_L = -90+climbing_rate*t1; % 3D
    % z_L = -90+10*sin(3*omega*t); % 3D
    % z_L = -90; %2D
    
    x_L_dot = r*omega*cos(omega*t);
    y_L_dot = -r*omega*sin(omega*t);
    z_L_dot = climbing_rate; % 3D
    % z_L_dot = 30*cos(3*omega*t); % 3D
    % z_L_dot = 0; % 2D
    y_L_dotdot = -r*omega^2*cos(omega*t);
    x_L_dotdot = -r*omega^2*sin(omega*t);
    course_L = atan2(y_L_dot,x_L_dot);
    course_L_dot = (y_L_dotdot*x_L_dot-x_L_dotdot*y_L_dot)/(x_L_dot^2+y_L_dot^2);
end

== matlab function Multi_FW_formation_control_wind/Virtual Leader Trajectory/Mixed trajectory(NED)/Switch Case Action Subsystem3/Circle trajectory(NED) ==
  data: x_L output; y_L output; z_L output; course_L output; z_L_dot output; course_L_dot output; r input; l input; Va_L input; t input; rs input
  function [x_L, y_L, z_L, course_L, z_L_dot, course_L_dot] = trajectory_generation(r,l,Va_L, t, rs)
    t1 = t - 2*rs;
    climbing_rate = 2; % 3D
    Va_Lp = sqrt(Va_L^2-climbing_rate^2);
    omega = Va_Lp/r; % rad/s
    x_L = -l/2+r*sin(omega*t);
    y_L = -l/2+r*cos(omega*t);
    z_L = -90-2*rs+climbing_rate*t1; % 3D
    % z_L = -90+10*sin(3*omega*t); % 3D
    % z_L = -90; %2D
    
    x_L_dot = r*omega*cos(omega*t);
    y_L_dot = -r*omega*sin(omega*t);
    z_L_dot = climbing_rate; % 3D
    % z_L_dot = 30*cos(3*omega*t); % 3D
    % z_L_dot = 0; % 2D

    x_L_dotdot = -r*omega^2*sin(omega*t);
    y_L_dotdot = -r*omega^2*cos(omega*t);
    course_L = atan2(y_L_dot,x_L_dot);
    course_L_dot = (y_L_dotdot*x_L_dot-x_L_dotdot*y_L_dot)/(x_L_dot^2+y_L_dot^2);
end

== matlab function Multi_FW_formation_control_wind/Virtual Leader Trajectory/Mixed trajectory(NED)/Switch Case Action Subsystem4/Line trajectory(NED) ==
  data: x_L output; y_L output; z_L output; course_L output; z_L_dot output; course_L_dot output; Va_L input; t input; r input; l input; rs input
function [x_L, y_L, z_L, course_L, z_L_dot, course_L_dot] = trajectory_generation(Va_L, t,r,l, rs)
    climbing_rate = 0; % 3D
    Va_Lp = sqrt(Va_L^2-climbing_rate^2);
    x_L = -l/2-r;    
    y_L = -l/2+Va_Lp*t*cos(0);
    % z_L = -90;
    z_L = -90; % 3D

    x_L_dot = 0;
    y_L_dot = Va_Lp*cos(0);
    % z_L_dot = 0;
    z_L_dot = climbing_rate; % 3D
    course_L = atan2(y_L_dot,x_L_dot);
    course_L_dot = 0;
end

== matlab function Multi_FW_formation_control_wind/Virtual Leader Trajectory/Mixed trajectory(NED)/Switch Case Action Subsystem5/Circle trajectory(NED) ==
  data: x_L output; y_L output; z_L output; course_L output; z_L_dot output; course_L_dot output; r input; l input; Va_L input; t input; rs input
  function [x_L, y_L, z_L, course_L, z_L_dot, course_L_dot] = trajectory_generation(r,l,Va_L, t, rs)
    t1 = t -3*rs;
    climbing_rate = -2; % 3D
    Va_Lp = sqrt(Va_L^2-climbing_rate^2);
    omega = Va_Lp/r; % rad/s
    x_L = -l/2+r*sin(omega*t);
    y_L = l/2+r*cos(omega*t);
    z_L = -90+climbing_rate*t1; % 3D
    % z_L = -90+10*sin(3*omega*t); % 3D
    % z_L = -90; %2D
    
    x_L_dot = r*omega*cos(omega*t);
    y_L_dot = -r*omega*sin(omega*t);
    z_L_dot = climbing_rate; % 3D
    % z_L_dot = 30*cos(3*omega*t); % 3D
    % z_L_dot = 0; % 2D

    x_L_dotdot = -r*omega^2*sin(omega*t);
    y_L_dotdot = -r*omega^2*cos(omega*t);
    course_L = atan2(y_L_dot,x_L_dot);
    course_L_dot = (y_L_dotdot*x_L_dot-x_L_dotdot*y_L_dot)/(x_L_dot^2+y_L_dot^2);
end

== matlab function Multi_FW_formation_control_wind/Virtual Leader Trajectory/Mixed trajectory(NED)/Switch Case Action Subsystem6/Line trajectory(NED) ==
  data: x_L output; y_L output; z_L output; course_L output; z_L_dot output; course_L_dot output; Va_L input; t input; r input; l input; rs input
function [x_L, y_L, z_L, course_L, z_L_dot, course_L_dot] = trajectory_generation(Va_L, t,r,l, rs)
    climbing_rate = 0; % 3D
    Va_Lp = sqrt(Va_L^2-climbing_rate^2);
    x_L = -l/2+Va_Lp*t*sin(pi/2);    
    y_L = l/2+r;
    % z_L = -90;
    z_L = -90-2*rs; % 3D

    x_L_dot = Va_Lp*sin(pi/2);
    y_L_dot = 0;
    % z_L_dot = 0;
    z_L_dot = climbing_rate; % 3D
    course_L = atan2(y_L_dot,x_L_dot);
    course_L_dot = 0;
end

== matlab function Multi_FW_formation_control_wind/Virtual Leader Trajectory/Mixed trajectory(NED)/Switch Case Action Subsystem7/Circle trajectory(NED) ==
  data: x_L output; y_L output; z_L output; course_L output; z_L_dot output; course_L_dot output; r input; l input; Va_L input; t input; rs input
  function [x_L, y_L, z_L, course_L, z_L_dot, course_L_dot] = trajectory_generation(r,l,Va_L, t, rs)
    t1 = t - 0*rs;
    climbing_rate = 2; % 3D descent
    Va_Lp = sqrt(Va_L^2-climbing_rate^2);
    omega = Va_Lp/r; % rad/s
    x_L = l/2+r*sin(omega*t);
    y_L = l/2+r*cos(omega*t);
    z_L = -90-2*rs+climbing_rate*t1; % 3D
    % z_L = -90+10*sin(3*omega*t); % 3D
    % z_L = -90; %2D
    
    x_L_dot = r*omega*cos(omega*t);
    y_L_dot = -r*omega*sin(omega*t);
    z_L_dot = climbing_rate; % 3D
    % z_L_dot = 30*cos(3*omega*t); % 3D
    % z_L_dot = 0; % 2D

    x_L_dotdot = -r*omega^2*sin(omega*t);
    y_L_dotdot = -r*omega^2*cos(omega*t);
    course_L = atan2(y_L_dot,x_L_dot);
    course_L_dot = (y_L_dotdot*x_L_dot-x_L_dotdot*y_L_dot)/(x_L_dot^2+y_L_dot^2);
end

== matlab function Multi_FW_formation_control_wind/Virtual Leader Trajectory/Mixed trajectory(NED)/MATLAB Function ==
  data: VL input; r input; rs output; l input; ls output
function [rs,ls] = fcn(VL,r,l)
    rs = r*2*pi/VL/4;
    ls = l/VL;
end

== matlab function Multi_FW_formation_control_wind/Virtual Leader Trajectory/Mixed trajectory(NED)/Switch Case Action Subsystem/Line trajectory(NED) ==
  data: x_L output; y_L output; z_L output; course_L output; z_L_dot output; course_L_dot output; Va_L input; t input; r input; l input
function [x_L, y_L, z_L, course_L, z_L_dot, course_L_dot] = trajectory_generation(Va_L, t,r,l)
    climbing_rate = 0; % 3D
    Va_Lp = sqrt(Va_L^2-climbing_rate^2);
    x_L = l/2+r;    
    y_L = l/2+Va_Lp*t*cos(-pi);
    % z_L = -90;
    z_L = -90+climbing_rate*t; % 3D
    x_L_dot = 0;
    y_L_dot = Va_Lp*cos(-pi);
    % z_L_dot = 0;
    z_L_dot = climbing_rate; % 3D
    course_L = atan2(y_L_dot,x_L_dot);
    course_L_dot = 0;
end

== matlab function Multi_FW_formation_control_wind/Virtual Leader Trajectory/Mixed trajectory(NED)/MATLAB Function1 ==
  data: rs input; ls input; offset output
function offset = fcn(rs,ls)
    offset = -ls+rs;
end

== matlab function Multi_FW_formation_control_wind/Virtual Leader Trajectory/Mixed trajectory(NED)/MATLAB Function2 ==
  data: rs input; ls input; offset output
function offset = fcn(rs,ls)
    offset = -ls-rs;
end

== matlab function Multi_FW_formation_control_wind/Virtual Leader Trajectory/Mixed trajectory(NED)/MATLAB Function3 ==
  data: rs input; ls input; offset output
function offset = fcn(rs,ls)
    offset = -2*ls+rs;
end

== matlab function Multi_FW_formation_control_wind/Virtual Leader Trajectory/Mixed trajectory(NED)/MATLAB Function4 ==
  data: rs input; ls input; offset output
function offset = fcn(rs,ls)
    offset = -2*ls-2*rs;
end

== matlab function Multi_FW_formation_control_wind/Virtual Leader Trajectory/Mixed trajectory(NED)/MATLAB Function5 ==
  data: rs input; ls input; offset output
function offset = fcn(rs,ls)
    offset = -3*ls+rs;
end

== matlab function Multi_FW_formation_control_wind/Virtual Leader Trajectory/Mixed trajectory(NED)/MATLAB Function6 ==
  data: rs input; ls input; offset output
function offset = fcn(rs,ls)
    offset = -3*ls-3*rs;
end

== matlab function Multi_FW_formation_control_wind/Virtual Leader Trajectory/Mixed trajectory(NED)/MATLAB Function7 ==
  data: rs input; ls input; offset output
function offset = fcn(rs,ls)
    offset = -4*ls-3*rs;
end

== matlab function Multi_FW_formation_control_wind/NED -> ENU 1 ==
  data: position_NED input; position_ENU output
function position_ENU = fcn(position_NED)
R_NED_ENU = [0 1 0;
             1 0 0;
             0 0 -1;];
position_ENU = R_NED_ENU* position_NED;
end

== matlab function Multi_FW_formation_control_wind/NED -> ENU 2 ==
  data: position_NED input; position_ENU output
function position_ENU = fcn(position_NED)
R_NED_ENU = [0 1 0;
             1 0 0;
             0 0 -1;];
position_ENU = R_NED_ENU* position_NED;
end

== matlab function Multi_FW_formation_control_wind/Virtual Leader Trajectory/Mixed trajectory(NED)/determine ==
  data: ca output; t input; rs input; ls input
function ca = case_determined(t, rs, ls)
    ca = 0;
    if t < ls
        ca = 1;
    elseif (t >= ls) & (t < ls + rs)
        ca = 2;
    elseif (t >= ls + rs) & (t < 2*ls + rs)
        ca = 3;
    elseif (t >= 2*ls + rs) & (t < 2*ls + 2*rs)
        ca = 4;
    elseif (t >= 2*ls + 2*rs) & (t < 3*ls + 2*rs)
        ca = 5;
    elseif (t >= 3*ls + 2*rs) & (t < 3*ls + 3*rs)
        ca = 6;
    elseif (t >= 3*ls + 3*rs) & (t < 4*ls + 3*rs)
        ca = 7;
    elseif (t >= 4*ls + 3*rs) & (t < 4*ls + 4*rs)
        ca = 8;
    end
end

== matlab function Multi_FW_formation_control_wind/NED -> ENU 3 ==
  data: position_NED input; position_ENU output
function position_ENU = fcn(position_NED)
R_NED_ENU = [0 1 0;
             1 0 0;
             0 0 -1;];
position_ENU = R_NED_ENU* position_NED;
end

== matlab function Multi_FW_formation_control_wind/Virtual Leader Trajectory/Circle trajectory(NED) ==
  data: x_L output; y_L output; z_L output; course_L output; z_L_dot output; course_L_dot output; r input; Va_L input; t input
  function [x_L, y_L, z_L, course_L, z_L_dot, course_L_dot] = trajectory_generation(r,Va_L, t)
    climbing_rate = -2; % 3D
    Va_Lp = sqrt(Va_L^2-climbing_rate^2);
    omega = Va_Lp/r; % rad/s
    x_L = r*cos(omega*t);
    y_L = r*sin(omega*t);
    z_L = -90+climbing_rate*t; % 3D
    % z_L = -90+10*sin(3*omega*t); % 3D
    % z_L = -90; %2D
    
    x_L_dot = -r*omega*sin(omega*t);
    y_L_dot = r*omega*cos(omega*t);
    z_L_dot = climbing_rate; % 3D
    % z_L_dot = 30*cos(3*omega*t); % 3D
    % z_L_dot = 0; % 2D
    x_L_dotdot = -r*omega^2*cos(omega*t);
    y_L_dotdot = -r*omega^2*sin(omega*t);
    course_L = atan2(y_L_dot,x_L_dot);
    course_L_dot = (y_L_dotdot*x_L_dot-x_L_dotdot*y_L_dot)/(x_L_dot^2+y_L_dot^2);
end

== matlab function Multi_FW_formation_control_wind/Virtual Leader Trajectory/Line trajectory(NED) ==
  data: Va_L input; dir input; x_L output; y_L output; z_L output; course_L output; z_L_dot output; course_L_dot output; t input
function [x_L, y_L, z_L, course_L, z_L_dot, course_L_dot] = trajectory_generation(Va_L,dir, t)
    climbing_rate = -2; % 3D
    Va_Lp = sqrt(Va_L^2-climbing_rate^2);
    x_L = Va_Lp*t*cos(dir);    
    y_L = Va_Lp*t*sin(dir);
    % z_L = -90;
    z_L = -90+climbing_rate*t; % 3D
    x_L_dot = Va_Lp*cos(dir);
    y_L_dot = Va_Lp*sin(dir);
    % z_L_dot = 0;
    z_L_dot = climbing_rate; % 3D
    course_L = atan2(y_L_dot,x_L_dot);
    course_L_dot = 0;
end

== matlab function Multi_FW_formation_control_wind/Virtual Leader Trajectory/Mixed trajectory(NED)/Switch Case Action Subsystem2/Line trajectory(NED) ==
  data: x_L output; y_L output; z_L output; course_L output; z_L_dot output; course_L_dot output; Va_L input; t input; r input; l input; rs input
function [x_L, y_L, z_L, course_L, z_L_dot, course_L_dot] = trajectory_generation(Va_L, t,r,l, rs)
    climbing_rate = 0; % 3D
    Va_Lp = sqrt(Va_L^2-climbing_rate^2);
    x_L = l/2+Va_Lp*t*sin(3/2*pi);    
    y_L = -l/2-r;
    % z_L = -90;
    z_L = -90-2*rs; % 3D
    x_L_dot = Va_Lp*sin(3/2*pi);
    y_L_dot = 0;
    % z_L_dot = 0;
    z_L_dot = climbing_rate; % 3D
    course_L = atan2(y_L_dot,x_L_dot);
    course_L_dot = 0;
end
